simulink model "SFENG_3K04_Ass1_Simulink"  (R2020a)
settings: Solver=FixedStepAuto  StartTime=0.0  StopTime=10.0  RelTol=1e-3  EnableMultiTasking=on
undefined symbols (not defined in the file or in its folder): D0, D1, D10, D11, D12, D13, D2, D3, D4, D5, D6, D7, D8, D9, PTA0, PTA1, PTA2, PTB23, PTB9, PTC16, PTC17, PTC2, PTC3, PTC4, PTD0, PTD1, PTD2, PTD3
libraries: frdmk64flib x15
settings Model: ExtModeTrigDuration=5  Creator=22538  LastModifiedBy=shivr
settings OptimizationCC: EnhancedBackFolding=on  PassReuseOutputArgsAs=Individual arguments  ZeroExternalMemoryAtStartup=off  ZeroInternalMemoryAtStartup=off  MaxStackSize=64  OptimizeBlockOrder=speed  DifferentSizesBufferReuse=on  OptimizationCustomize=off  EfficientTunableParamExpr=on
settings DebuggingCC: ParameterTunabilityLossMsg=error
settings HardwareCC: ProdBitPerPointer=32  ProdBitPerSizeT=32  ProdBitPerPtrDiffT=32  ProdLargestAtomicInteger=Long  ProdLargestAtomicFloat=Double  ProdWordSize=32  ProdHWDeviceType=ARM Compatible->ARM Cortex
settings SFSimCC: MATLABDynamicMemAlloc=off
settings RTWCC: SystemTargetFile=ert.tlc  HardwareBoard=NXP FRDM-K64F  TemplateMakefile=ert_default_tmf  Toolchain=GNU Tools for ARM Embedded Processors
settings CodeAppCC: ForceParamTrailComments=on  IgnoreCustomStorageClasses=off  OperatorAnnotations=on  SimulinkDataObjDesc=on  SFDataObjDesc=on  InsertBlockDesc=on

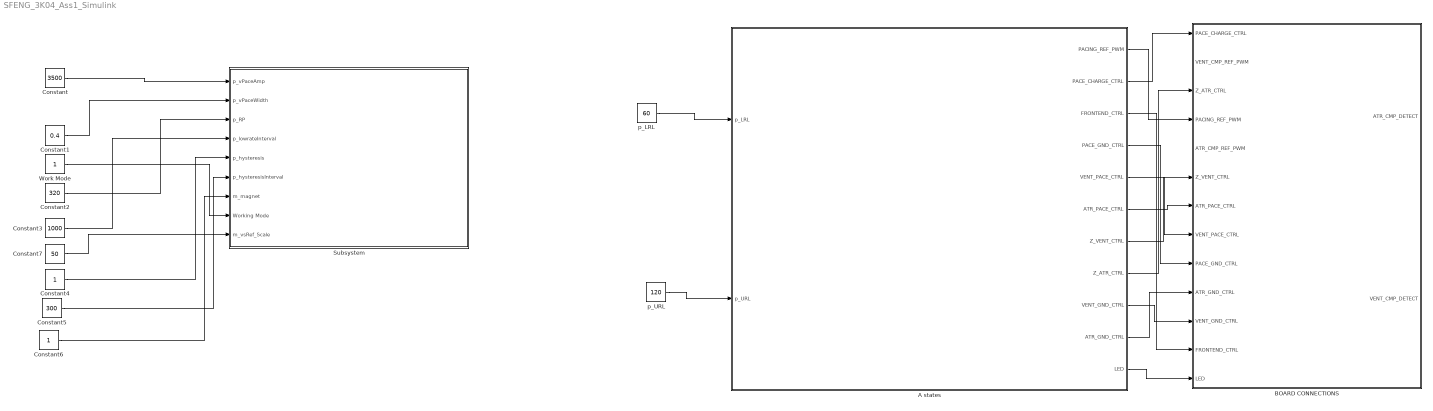
== system SFENG_3K04_Ass1_Simulink ==
  A states : Subsystem
  BOARD CONNECTIONS : Subsystem
  Constant : Constant  Value=3500  OutMin=500  OutMax=7000
  Constant1 : Constant  Value=0.4
  Constant2 : Constant  Value=320
  Constant3 : Constant  Value=1000
  Constant4 : Constant
  Constant5 : Constant  Value=300
  Constant6 : Constant
  Constant7 : Constant  Value=50
  Subsystem : Subsystem
  Work Mode : Constant
  p_LRL : Constant  Value=60
  p_URL : Constant  Value=120
  wires:
  Constant/1 -> Subsystem/1(p_vPaceAmp)
  Constant1/1 -> Subsystem/2(p_vPaceWidth)
  Constant2/1 -> Subsystem/3(p_RP)
  Constant3/1 -> Subsystem/4(p_lowrateInterval)
  Constant4/1 -> Subsystem/5(p_hysteresis)
  Constant5/1 -> Subsystem/6(p_hysteresisInterval)
  Constant6/1 -> Subsystem/7(m_magnet)
  Constant7/1 -> Subsystem/9(m_vsRef_Scale)
  Work Mode/1 -> Subsystem/8(Working Mode)
  A states/11(LED) -> BOARD CONNECTIONS/13(LED)
  A states/1(PACING_REF_PWM) -> BOARD CONNECTIONS/4(PACING_REF_PWM)
  A states/6(ATR_PACE_CTRL) -> BOARD CONNECTIONS/7(ATR_PACE_CTRL)
  A states/2(PACE_CHARGE_CTRL) -> BOARD CONNECTIONS/1(PACE_CHARGE_CTRL)
  p_URL/1 -> A states/2(p_URL)
  A states/3(FRONTEND_CTRL) -> BOARD CONNECTIONS/12(FRONTEND_CTRL)
  A states/5(VENT_PACE_CTRL) -> BOARD CONNECTIONS/8(VENT_PACE_CTRL)
  A states/8(Z_ATR_CTRL) -> BOARD CONNECTIONS/3(Z_ATR_CTRL)
  A states/7(Z_VENT_CTRL) -> BOARD CONNECTIONS/6(Z_VENT_CTRL)
  A states/4(PACE_GND_CTRL) -> BOARD CONNECTIONS/9(PACE_GND_CTRL)
  p_LRL/1 -> A states/1(p_LRL)
  A states/10(ATR_GND_CTRL) -> BOARD CONNECTIONS/10(ATR_GND_CTRL)
  A states/9(VENT_GND_CTRL) -> BOARD CONNECTIONS/11(VENT_GND_CTRL)

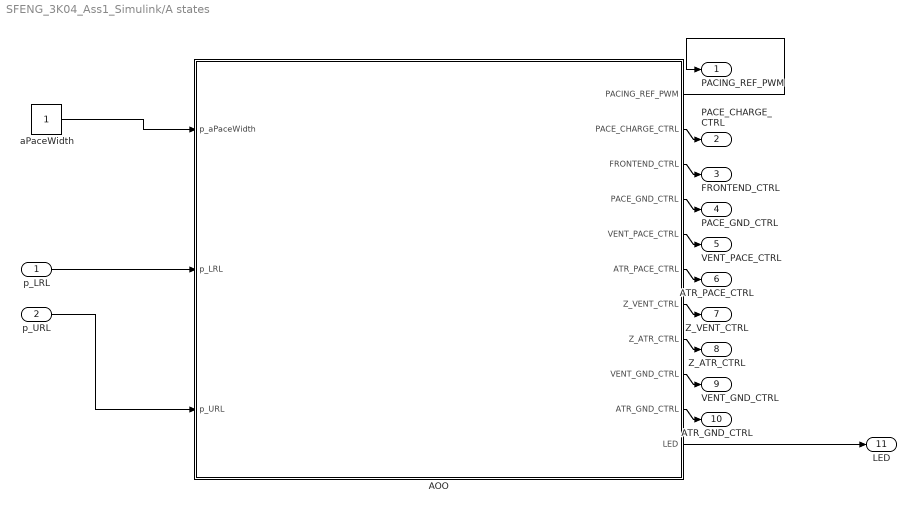
== system SFENG_3K04_Ass1_Simulink/A states ==
  p_LRL : Inport
  p_URL : Inport  Port=2
  AOO : Stateflow chart  TreatAsAtomicUnit=on
  aPaceWidth : Constant
  PACING_REF_PWM : Outport
  PACE_CHARGE_CTRL : Outport  Port=2
  FRONTEND_CTRL : Outport  Port=3
  PACE_GND_CTRL : Outport  Port=4
  VENT_PACE_CTRL : Outport  Port=5
  ATR_PACE_CTRL : Outport  Port=6
  Z_VENT_CTRL : Outport  Port=7
  Z_ATR_CTRL : Outport  Port=8
  VENT_GND_CTRL : Outport  Port=9
  ATR_GND_CTRL : Outport  Port=10
  LED : Outport  Port=11
  wires:
  aPaceWidth/1 -> AOO/1(p_aPaceWidth)
  AOO/5(VENT_PACE_CTRL) -> VENT_PACE_CTRL/1
  AOO/3(FRONTEND_CTRL) -> FRONTEND_CTRL/1
  AOO/1(PACING_REF_PWM) -> PACING_REF_PWM/1
  AOO/6(ATR_PACE_CTRL) -> ATR_PACE_CTRL/1
  AOO/7(Z_VENT_CTRL) -> Z_VENT_CTRL/1
  AOO/4(PACE_GND_CTRL) -> PACE_GND_CTRL/1
  AOO/8(Z_ATR_CTRL) -> Z_ATR_CTRL/1
  AOO/2(PACE_CHARGE_CTRL) -> PACE_CHARGE_CTRL/1
  AOO/9(VENT_GND_CTRL) -> VENT_GND_CTRL/1
  AOO/10(ATR_GND_CTRL) -> ATR_GND_CTRL/1
  AOO/11(LED) -> LED/1
  p_LRL/1 -> AOO/2(p_LRL)
  p_URL/1 -> AOO/3(p_URL)

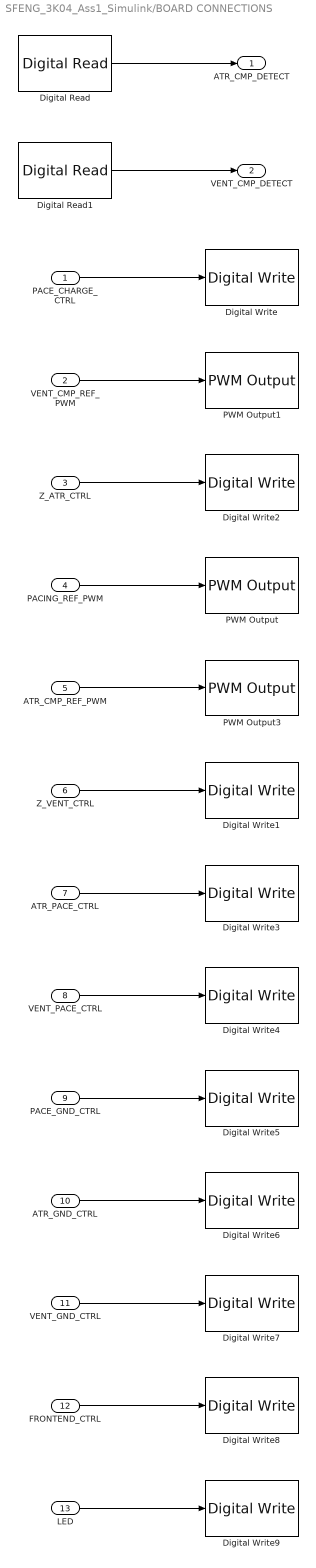
== system SFENG_3K04_Ass1_Simulink/BOARD CONNECTIONS ==
  PACE_CHARGE_CTRL : Inport
  VENT_CMP_REF_PWM : Inport  Port=2
  Z_ATR_CTRL : Inport  Port=3
  PACING_REF_PWM : Inport  Port=4
  ATR_CMP_REF_PWM : Inport  Port=5
  Z_VENT_CTRL : Inport  Port=6
  ATR_PACE_CTRL : Inport  Port=7
  VENT_PACE_CTRL : Inport  Port=8
  PACE_GND_CTRL : Inport  Port=9
  ATR_GND_CTRL : Inport  Port=10
  VENT_GND_CTRL : Inport  Port=11
  FRONTEND_CTRL : Inport  Port=12
  LED : Inport  Port=13
  Digital Read : frdmk64flib/Digital Read  Whichpin=PTC16 (D0)  SampleTime=-1
  Digital Read1 : frdmk64flib/Digital Read  Whichpin=PTC17 (D1)  SampleTime=-1
  Digital Write : frdmk64flib/Digital Write  Whichpin=PTB9 (D2)
  Digital Write1 : frdmk64flib/Digital Write  Whichpin=PTC3 (D7)
  Digital Write2 : frdmk64flib/Digital Write  Whichpin=PTB23 (D4)
  Digital Write3 : frdmk64flib/Digital Write  Whichpin=PTA0 (D8)
  Digital Write4 : frdmk64flib/Digital Write  Whichpin=PTC4 (D9)
  Digital Write5 : frdmk64flib/Digital Write  Whichpin=PTD0 (D10)
  Digital Write6 : frdmk64flib/Digital Write  Whichpin=PTD2 (D11)
  Digital Write7 : frdmk64flib/Digital Write  Whichpin=PTD3 (D12)
  Digital Write8 : frdmk64flib/Digital Write  Whichpin=PTD1 (D13)
  Digital Write9 : frdmk64flib/Digital Write  Whichpin=RED_LED
  PWM Output : frdmk64flib/PWM Output  Whichpin=PTA2 (D5)  InitialFrequency=2000  InitialDutyCycle=0
  PWM Output1 : frdmk64flib/PWM Output  Whichpin=PTA1 (D3)  InitialFrequency=2000  InitialDutyCycle=0
  PWM Output3 : frdmk64flib/PWM Output  Whichpin=PTC2 (D6)  InitialFrequency=2000  InitialDutyCycle=100
  ATR_CMP_DETECT : Outport
  VENT_CMP_DETECT : Outport  Port=2
  wires:
  Digital Read/1 -> ATR_CMP_DETECT/1
  Digital Read1/1 -> VENT_CMP_DETECT/1
  VENT_CMP_REF_PWM/1 -> PWM Output1/1
  PACE_CHARGE_CTRL/1 -> Digital Write/1
  Z_ATR_CTRL/1 -> Digital Write2/1
  PACING_REF_PWM/1 -> PWM Output/1
  ATR_CMP_REF_PWM/1 -> PWM Output3/1
  Z_VENT_CTRL/1 -> Digital Write1/1
  ATR_PACE_CTRL/1 -> Digital Write3/1
  VENT_PACE_CTRL/1 -> Digital Write4/1
  PACE_GND_CTRL/1 -> Digital Write5/1
  ATR_GND_CTRL/1 -> Digital Write6/1
  VENT_GND_CTRL/1 -> Digital Write7/1
  FRONTEND_CTRL/1 -> Digital Write8/1
  LED/1 -> Digital Write9/1

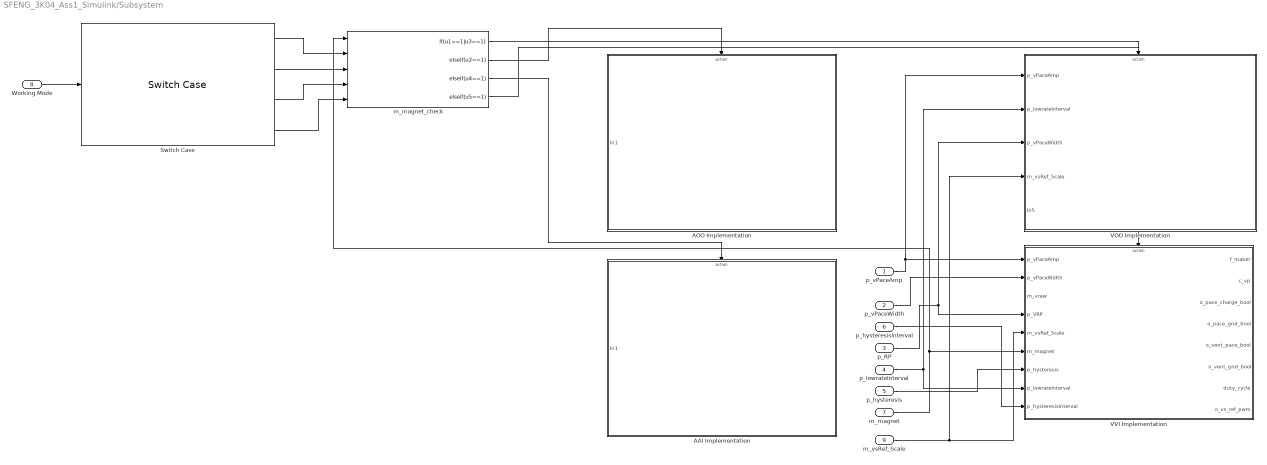
== system SFENG_3K04_Ass1_Simulink/Subsystem ==
  p_vPaceAmp : Inport
  p_vPaceWidth : Inport  Port=2
  p_RP : Inport  Port=3
  p_lowrateInterval : Inport  Port=4
  p_hysteresis : Inport  Port=5
  p_hysteresisInterval : Inport  Port=6
  m_magnet : Inport  Port=7
  Working Mode : Inport  Port=8
  m_vsRef_Scale : Inport  Port=9
  AAI Implementation : Subsystem
  AOO Implementation : Subsystem
  Switch Case : SwitchCase  CaseConditions={1,2,3,4}  ShowDefaultCase=off
  VOO Implementation : Subsystem
  VVI Implementation : Subsystem
  m_magnet_check : If  NumInputs=5  IfExpression=u1==1|u3==1  ElseIfExpressions=u2==1,u4==1,u5==1  ShowElse=off
  wires:
  p_vPaceAmp/1 -> VOO Implementation/1(p_vPaceAmp), VVI Implementation/1(p_vPaceAmp)
  p_vPaceWidth/1 -> VVI Implementation/2(p_vPaceWidth)
  p_RP/1 -> VOO Implementation/3(p_vPaceWidth), VVI Implementation/4(p_VRP)
  m_magnet/1 -> m_magnet_check/1, VVI Implementation/6(m_magnet)
  p_hysteresis/1 -> VVI Implementation/7(p_hysteresis)
  p_lowrateInterval/1 -> VOO Implementation/2(p_lowrateInterval), VVI Implementation/8(p_lowrateInterval)
  p_hysteresisInterval/1 -> VVI Implementation/9(p_hysteresisInterval)
  Working Mode/1 -> Switch Case/1
  Switch Case/1 -> m_magnet_check/2
  Switch Case/2 -> m_magnet_check/3
  Switch Case/3 -> m_magnet_check/4
  Switch Case/4 -> m_magnet_check/5
  m_magnet_check/2 -> AOO Implementation/Action
  m_magnet_check/1 -> VOO Implementation/Action
  m_magnet_check/3 -> AAI Implementation/Action
  m_magnet_check/4 -> VVI Implementation/Action
  m_vsRef_Scale/1 -> VOO Implementation/4(m_vsRef_Scale), VVI Implementation/5(m_vsRef_Scale)

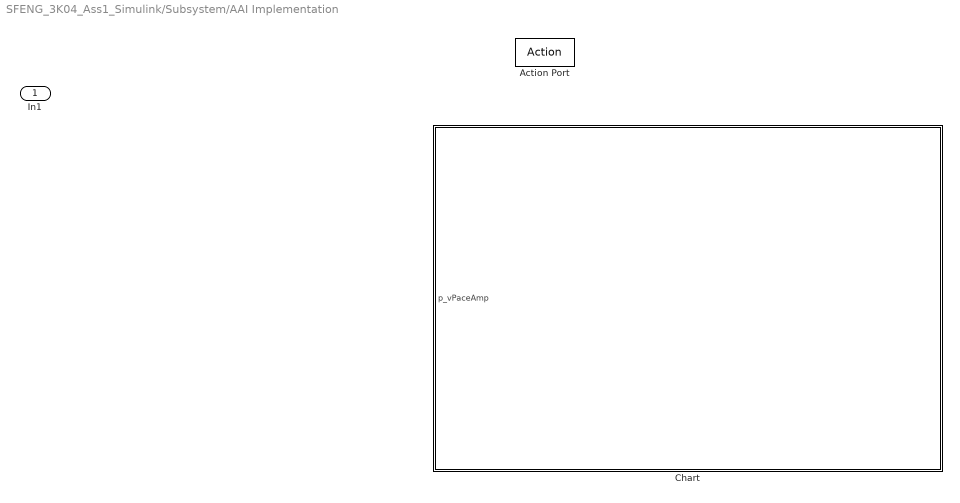
== system SFENG_3K04_Ass1_Simulink/Subsystem/AAI Implementation ==
  In1 : Inport
  Action Port : ActionPort  ActionPortLabel=elseif(u4==1)
  Chart : Stateflow chart  TreatAsAtomicUnit=on

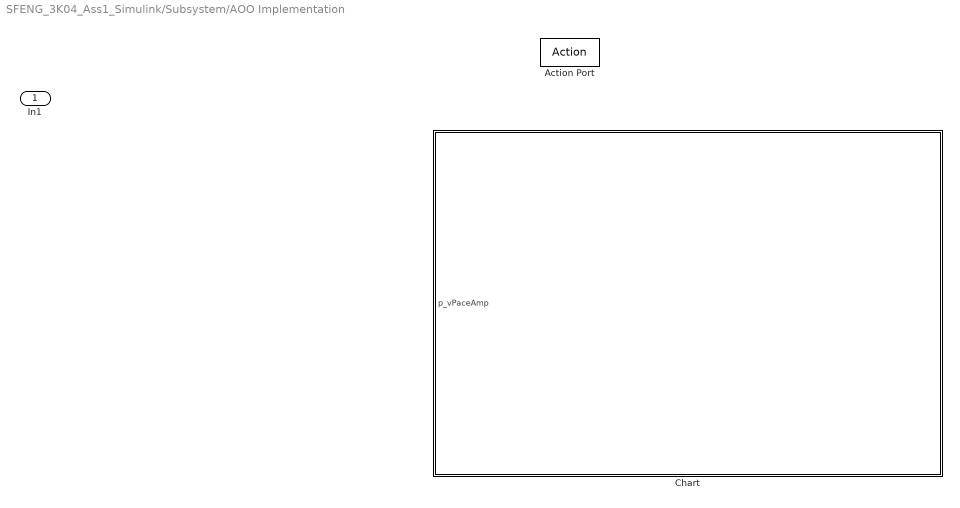
== system SFENG_3K04_Ass1_Simulink/Subsystem/AOO Implementation ==
  In1 : Inport
  Action Port : ActionPort  ActionPortLabel=elseif(u2==1)
  Chart : Stateflow chart  TreatAsAtomicUnit=on

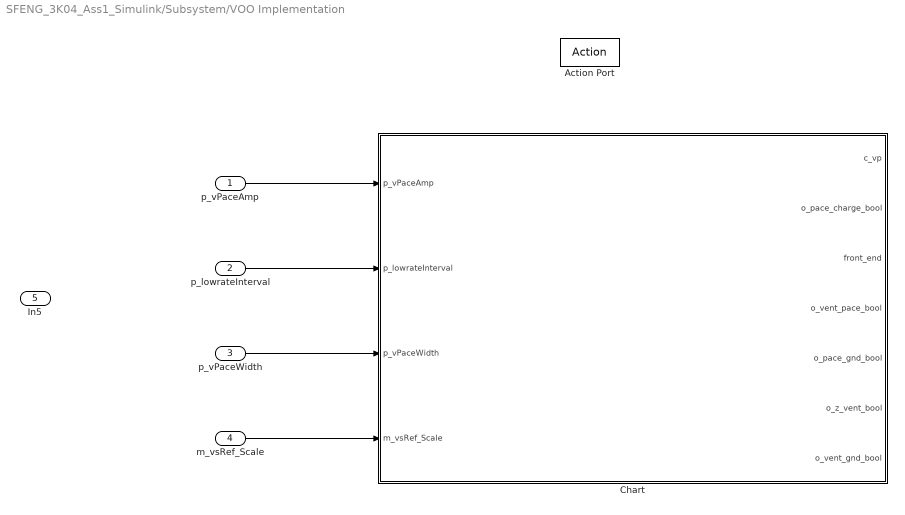
== system SFENG_3K04_Ass1_Simulink/Subsystem/VOO Implementation ==
  p_vPaceAmp : Inport
  p_lowrateInterval : Inport  Port=2
  p_vPaceWidth : Inport  Port=3
  m_vsRef_Scale : Inport  Port=4
  In5 : Inport  Port=5
  Action Port : ActionPort  ActionPortLabel=if(u1==1|u3==1)
  Chart : Stateflow chart  TreatAsAtomicUnit=on
  wires:
  p_vPaceAmp/1 -> Chart/1(p_vPaceAmp)
  p_lowrateInterval/1 -> Chart/2(p_lowrateInterval)
  p_vPaceWidth/1 -> Chart/3(p_vPaceWidth)
  m_vsRef_Scale/1 -> Chart/4(m_vsRef_Scale)

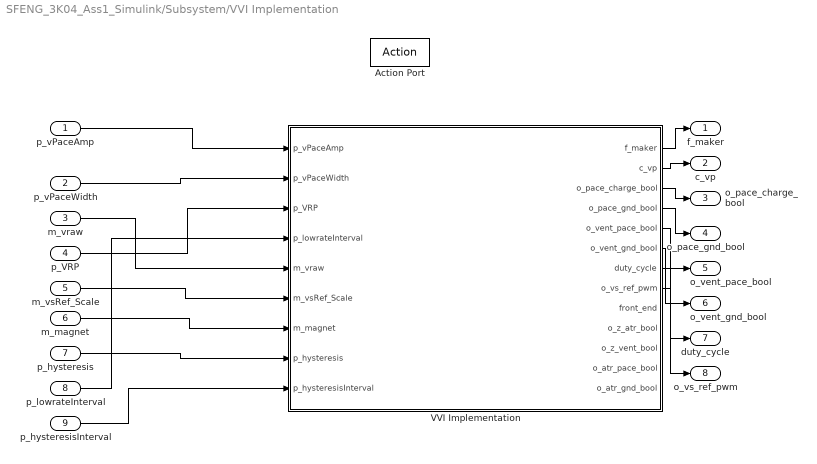
== system SFENG_3K04_Ass1_Simulink/Subsystem/VVI Implementation ==
  p_vPaceAmp : Inport
  p_vPaceWidth : Inport  Port=2
  m_vraw : Inport  Port=3
  p_VRP : Inport  Port=4
  m_vsRef_Scale : Inport  Port=5
  m_magnet : Inport  Port=6
  p_hysteresis : Inport  Port=7
  p_lowrateInterval : Inport  Port=8
  p_hysteresisInterval : Inport  Port=9
  Action Port : ActionPort  ActionPortLabel=elseif(u5==1)
  VVI Implementation : Stateflow chart  TreatAsAtomicUnit=on
  f_maker : Outport
  c_vp : Outport  Port=2
  o_pace_charge_bool : Outport  Port=3
  o_pace_gnd_bool : Outport  Port=4
  o_vent_pace_bool : Outport  Port=5
  o_vent_gnd_bool : Outport  Port=6
  duty_cycle : Outport  Port=7
  o_vs_ref_pwm : Outport  Port=8
  wires:
  m_vsRef_Scale/1 -> VVI Implementation/6(m_vsRef_Scale)
  m_magnet/1 -> VVI Implementation/7(m_magnet)
  VVI Implementation/8(o_vs_ref_pwm) -> o_vs_ref_pwm/1
  VVI Implementation/1(f_maker) -> f_maker/1
  VVI Implementation/2(c_vp) -> c_vp/1
  VVI Implementation/7(duty_cycle) -> duty_cycle/1
  p_vPaceWidth/1 -> VVI Implementation/2(p_vPaceWidth)
  VVI Implementation/6(o_vent_gnd_bool) -> o_vent_gnd_bool/1
  VVI Implementation/5(o_vent_pace_bool) -> o_vent_pace_bool/1
  p_hysteresisInterval/1 -> VVI Implementation/9(p_hysteresisInterval)
  VVI Implementation/3(o_pace_charge_bool) -> o_pace_charge_bool/1
  p_hysteresis/1 -> VVI Implementation/8(p_hysteresis)
  m_vraw/1 -> VVI Implementation/5(m_vraw)
  VVI Implementation/4(o_pace_gnd_bool) -> o_pace_gnd_bool/1
  p_lowrateInterval/1 -> VVI Implementation/4(p_lowrateInterval)
  p_vPaceAmp/1 -> VVI Implementation/1(p_vPaceAmp)
  p_VRP/1 -> VVI Implementation/3(p_VRP)

== stateflow chart SFENG_3K04_Ass1_Simulink/Subsystem/AAI Implementation/Chart ==
  state ?
  (default) -> ?
  data: p_vPaceAmp input [500..7000]

== stateflow chart SFENG_3K04_Ass1_Simulink/A states/AOO ==
  note: AOO
  state Pace
    entry:
    PACE_CHARGE_CTRL = false; %stop charging
    PACE_GND_CTRL = true;
    ATR_PACE_CTRL = true;
    ATR_GND_CTRL = false;
    Z_ATR_CTRL = false;
    Z_VENT_CTRL = false;
    VENT_GND_CTRL = false;
    VENT_PACE_CTRL = false;
    LED =true;
    %add LED as well
  state Prep
    entry:
    FRONTEND_CTRL=false; %sensing off
    %start charging C22
    ATR_PACE_CTRL = false;       %1
    VENT_PACE_CTRL = false;      %2
    PACING_REF_PWM = (Atrial_Amplitude/5) * 100; %3
    PACE_CHARGE_CTRL = true;  %4
    %discharge blocking (combined state)
    PACE_GND_CTRL = false; %
    Z_ATR_CTRL= false;
    Z_VENT_CTRL=false;
    %ATR_PACE_CTRL = false;
    ATR_GND_CTRL = true;
    VENT_GND_CTRL = false;
  (default) -> Prep
  Prep -> Pace : [after(60000/p_LRL-p_aPaceWidth, msec)]
  Pace -> Prep : [after(p_aPaceWidth, msec)]
  data: PACING_REF_PWM output; P_aPaceAmp parameter; PACE_CHARGE_CTRL output; FRONTEND_CTRL output; PACE_GND_CTRL output; VENT_PACE_CTRL output; ATR_PACE_CTRL output; Z_VENT_CTRL output; Z_ATR_CTRL output; VENT_GND_CTRL output; ATR_GND_CTRL output; LED output; p_aPaceWidth input; p_LRL input; p_URL input

== stateflow chart SFENG_3K04_Ass1_Simulink/Subsystem/VOO Implementation/Chart ==
  state VOO_Pace_State
    entry:
    c_vp=p_vPaceAmp;
    o_vent_pace_bool=true;
    o_vent_gnd_bool=false;
    o_pace_gnd_bool=true;
    o_pace_charge_bool=false;
    o_z_vent_bool=true;
  state VOO_Prep_State
    entry:
    front_end=true;
    o_pace_charge_bool=true;
    o_vent_pace_bool=false;
    o_pace_gnd_bool=true;
    o_vent_gnd_bool=true;
    o_z_vent_bool=false;
    c_vp=0;
  (default) -> VOO_Prep_State
  VOO_Prep_State -> VOO_Pace_State : [after(60000.0/p_lowrateInterval - p_vPaceWidth,msec)]
  VOO_Pace_State -> VOO_Prep_State : [after(p_vPaceWidth,msec)]
  data: p_vPaceAmp input [500..7000]; p_lowrateInterval input [343..2000]; p_vPaceWidth input [0.1..1.9]; m_vsRef_Scale input; c_vp output; o_pace_charge_bool output; front_end output; o_vent_pace_bool output; o_pace_gnd_bool output; o_z_vent_bool output; o_vent_gnd_bool output

== stateflow chart SFENG_3K04_Ass1_Simulink/Subsystem/AOO Implementation/Chart ==
  state ?
  (default) -> ?
  data: p_vPaceAmp input [500..7000]

== stateflow chart SFENG_3K04_Ass1_Simulink/Subsystem/VVI Implementation/VVI Implementation ==
  state VVI_Prep_State
    entry:
    front_end=true;
    o_vent_pace_bool=false;
    o_vent_gnd_bool=false;
    o_pace_charge_bool=true;
    o_pace_gnd_bool=true;
    o_z_vent_bool=false;
  state VVI_Pace_State
    entry:
    front_end=true;
    o_vent_pace_bool=true;
    o_vent_gnd_bool=true;
    o_pace_charge_bool=false;
    o_pace_gnd_bool=false;
    o_z_vent_bool=false;
  (default) -> VVI_Prep_State
  VVI_Prep_State -> VVI_Pace_State : [after((60000-(p_lowrateInterval*p_vPaceAmp))/p_lowrateInterval)]
  VVI_Pace_State -> VVI_Prep_State
  data: p_vPaceAmp input [500..7000]; p_vPaceWidth input double [0.1..1.9]; p_VRP input [150..500]; p_lowrateInterval input [343..2000]; m_vraw input double [5000.0..0.0]; m_vsRef_Scale input boolean [0..1]; m_magnet input boolean [0..1]; p_hysteresis input boolean [0..1]; p_hysteresisInterval input [343..2000]; f_maker output; c_vp output; o_pace_charge_bool output boolean [0..1]; o_pace_gnd_bool output boolean [0..1]; o_vent_pace_bool output boolean [0..1]; o_vent_gnd_bool output boolean [0..1]; duty_cycle output; o_vs_ref_pwm output; front_end output boolean; o_z_atr_bool output boolean; o_z_vent_bool output boolean; o_atr_pace_bool output boolean; o_atr_gnd_bool output boolean
